simulink model "BFnominale"  (R2017b)
settings: Solver=VariableStepAuto  StartTime=0.0  StopTime=100.0  RelTol=1e-3
settings Model: Creator=t.lopes  LastModifiedBy=t.lopes

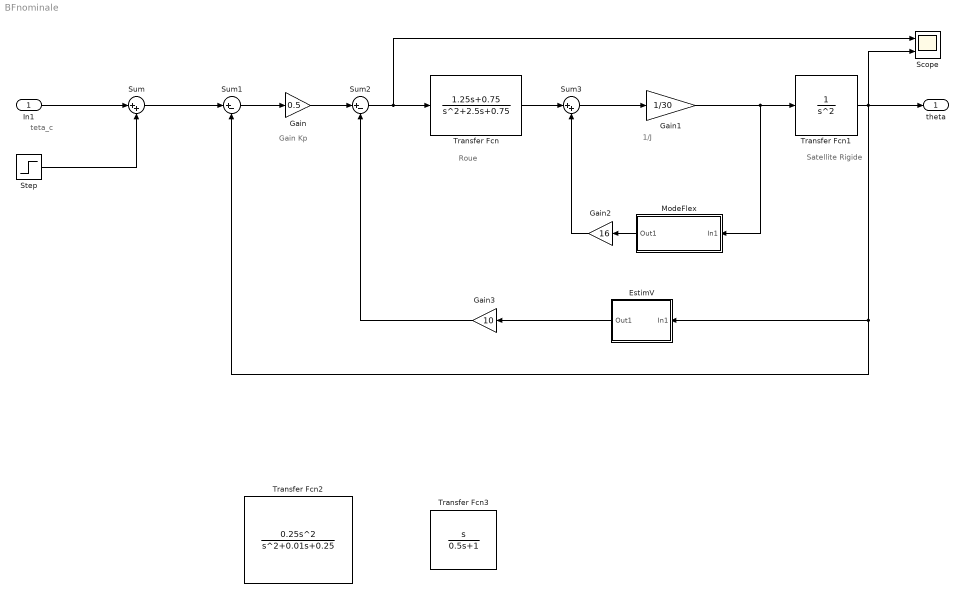
== system BFnominale ==
  note: Roue
  note: Satellite Rigide
  note: Gain Kp
  note: 1/J
  note: teta_c
  In1 : Inport
  EstimV : Subsystem
  Gain : Gain  Gain=0.5
  Gain1 : Gain  Gain=1/30
  Gain2 : Gain  Gain=16
  Gain3 : Gain  Gain=10
  ModeFlex : Subsystem
  Scope : Scope  NumInputPorts=2
  Step : Step  After=pi/180  SampleTime=0
  Sum : Sum  Inputs=|++
  Sum1 : Sum  Inputs=|+-
  Sum2 : Sum  Inputs=|+-
  Sum3 : Sum  Inputs=|++
  Transfer Fcn : TransferFcn  Numerator=[1.25 0.75]  Denominator=[1 2.5 0.75]
  Transfer Fcn1 : TransferFcn  Denominator=[1 0 0]
  Transfer Fcn2 : TransferFcn  Numerator=[0.25 0 0]  Denominator=[1 0.01 0.25]
  Transfer Fcn3 : TransferFcn  Numerator=[1 0]  Denominator=[0.5 1]
  "theta " : Outport
  wires:
  Step/1 -> Sum/2
  In1/1 -> Sum/1
  Sum/1 -> Sum1/1
  Gain3/1 -> Sum2/2
  Sum1/1 -> Gain/1
  Gain/1 -> Sum2/1
  Sum2/1 -> Scope/1, Transfer Fcn/1
  Transfer Fcn/1 -> Sum3/1
  Sum3/1 -> Gain1/1
  ModeFlex/1(Out1) -> Gain2/1
  Gain1/1 -> ModeFlex/1(In1), Transfer Fcn1/1
  Gain2/1 -> Sum3/2
  EstimV/1(Out1) -> Gain3/1
  Transfer Fcn1/1 -> Scope/2, "theta "/1, EstimV/1(In1), Sum1/2

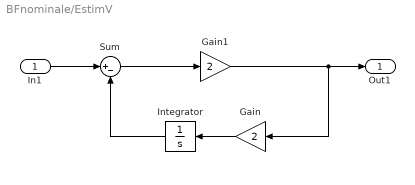
== system BFnominale/EstimV ==
  In1 : Inport
  Gain : Gain  Gain=2
  Gain1 : Gain  Gain=2
  Integrator : Integrator
  Sum : Sum  Inputs=|+-
  Out1 : Outport
  wires:
  In1/1 -> Sum/1
  Integrator/1 -> Sum/2
  Gain/1 -> Integrator/1
  Sum/1 -> Gain1/1
  Gain1/1 -> Out1/1, Gain/1

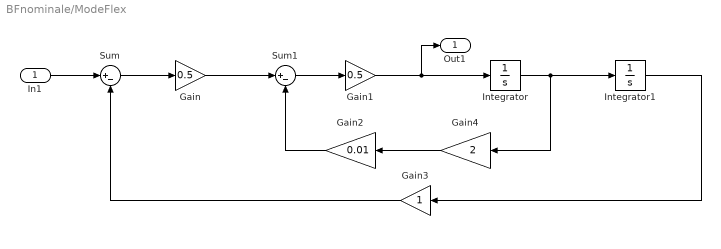
== system BFnominale/ModeFlex ==
  In1 : Inport
  Gain : Gain  Gain=0.5
  Gain1 : Gain  Gain=0.5
  Gain2 : Gain  Gain=0.01
  Gain3 : Gain
  Gain4 : Gain  Gain=2
  Integrator : Integrator
  Integrator1 : Integrator
  Sum : Sum  Inputs=|+-
  Sum1 : Sum  Inputs=|+-
  Out1 : Outport
  wires:
  In1/1 -> Sum/1
  Sum/1 -> Gain/1
  Gain/1 -> Sum1/1
  Gain2/1 -> Sum1/2
  Sum1/1 -> Gain1/1
  Gain1/1 -> Out1/1, Integrator/1
  Integrator1/1 -> Gain3/1
  Integrator/1 -> Gain4/1, Integrator1/1
  Gain3/1 -> Sum/2
  Gain4/1 -> Gain2/1
